simulink model "ElecTorqueCalculation"  (R2025b)
settings: Solver=VariableStepAuto  StartTime=0.0  StopTime=10.0  RelTol=1e-3
settings Model: Creator=jff_1  LastModifiedBy=jff_1

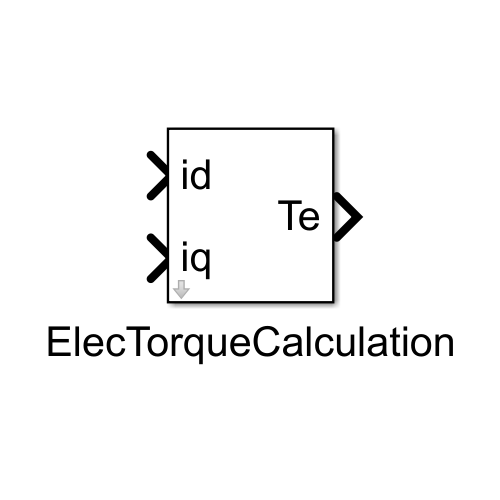
[thumbnail: Simulink's stored preview of the top-level diagram]
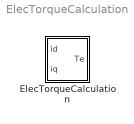
== system ElecTorqueCalculation ==
  ElecTorqueCalculation : Subsystem  mask{Pn=0, K=0, flux=0}
      mask prompts: Pn "极对数Pn"; K "Ld-Lq"; flux "磁链flux"
      mask help:
      | 该封装用于计算电磁转矩（Te），并根据输入的 d 轴电流（id）和 q 轴电流（iq）通过相应的公式进行计算。此模型根据给定的常见电机参数（如极对数、Ld-Lq 和磁链 flux）来推导电磁转矩的输出。
      |
      | 输入：
      |
      | id：d 轴电流（单位：A）
      |
      | iq：q 轴电流（单位：A）
      |
      | 输出：
      |
      | Te：电磁转矩（单位：Nm）
      |
      | 参数：
      |
      | 极对数 Pn：电机的极对数，通常取值如 2 或 4（具体根据电机设计而定）
      |
      | Ld-Lq：d 轴和 q 轴的电感差（单位：H）
      |
      | 磁链 flux：电机的磁链，通常由电机厂家提供或计算。
      |
      | 使用说明：
      |
      | 将 id 和 iq 输入到该模块，设置相关参数（Pn、Ld-Lq 和 flux），然后获取计算出的电磁转矩 Te。
      |
      | 该模块可以集成到更大的电机控制仿真模型中，用于估算电机转矩。
      mask Help:
      | 帮助：
      | 
      | 极对数 Pn：通常是 2 或 4，取决于电机的设计。
      | 
      | Ld-Lq：这两个电感值常见于永磁同步电机（PMSM），具体值依赖于电机参数。
      | 
      | 磁链 flux：磁链值根据电机设计参数给出，可由测试获得。
      mask DialogControl ParameterGroupVar Prompt: 参数
      mask Display:
      | % 输入标签
      | port_label('input', 1, 'id');
      | port_label('input', 2, 'iq');
      | 
      | % 输出标签
      | port_label('output', 1, 'Te');

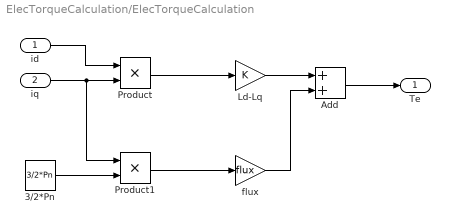
== system ElecTorqueCalculation/ElecTorqueCalculation ==
  id : Inport
  iq : Inport  Port=2
  3/2*Pn : Constant  Value=3/2*Pn
  Add : Sum
  Ld-Lq : Gain  Gain=K
  Product : Product
  Product1 : Product
  flux : Gain  Gain=flux
  Te : Outport
  wires:
  id/1 -> Product/1
  Product/1 -> Ld-Lq/1
  3/2*Pn/1 -> Product1/2
  Ld-Lq/1 -> Add/1
  Add/1 -> Te/1
  Product1/1 -> flux/1
  flux/1 -> Add/2
  iq/1 -> Product1/1, Product/2
